simulink model "simulink_model"  (R2019b)
settings: Solver=ode15s  StartTime=0.0  StopTime=sim_time  FixedStep=1e-5
values from neighbouring files (symbols this model uses):
  A_t = 2000*eye(n)    [config_2R.m]    (also in config_3R.m)
  B2 = -Jinv    [computegains.m]
  B_t = eye(n)    [computegains.m]
  J = diag(rg.^2 .* Im_zz)    [model_2R.m]    (also in model_3R.m)
  Jinv = inv(J)    [computegains.m]
  K = diag(k_el)    [model_2R.m]    (also in model_3R.m)
  K1_t = lyap(A_t,Q_t)    [config_2R.m]    (also in config_3R.m)
  K2_t = 2000*eye(n)    [config_2R.m]    (also in config_3R.m)
  K_ctr = K_ctr*T_ctr    [computegains.m]
  K_ctr2 = -place(At,Bt,pls_ctr2)    [computegains.m]
  Ka_t = -10000*eye(n)    [config_2R.m]    (also in config_3R.m)
  n = 3    [simulation.m]
  x0 = [-pi/2 0   , 0 0 , -pi/2 0 , 0 0]    [config_2R.m]    (also in config_3R.m = [0 pi/2 0 , 0 0 0 , 0 pi/2 0 , 0 0 0])
  x0_hat = [x0(1) x0(2) , 0 0   , 0 0  ,   0 0]    [config_2R.m]    (also in config_3R.m = [x0(1) x0(2) x0(3) , 0 0 0 , 0 0 0 , 0 0 0])
undefined symbols (not defined in the file or in its folder): F_fun, Q1_fun, Q2_fun, Q_fun
settings Model: Creator=pietro  LastModifiedBy=pietro
settings SolverCC: MaxConsecutiveMinStep=10

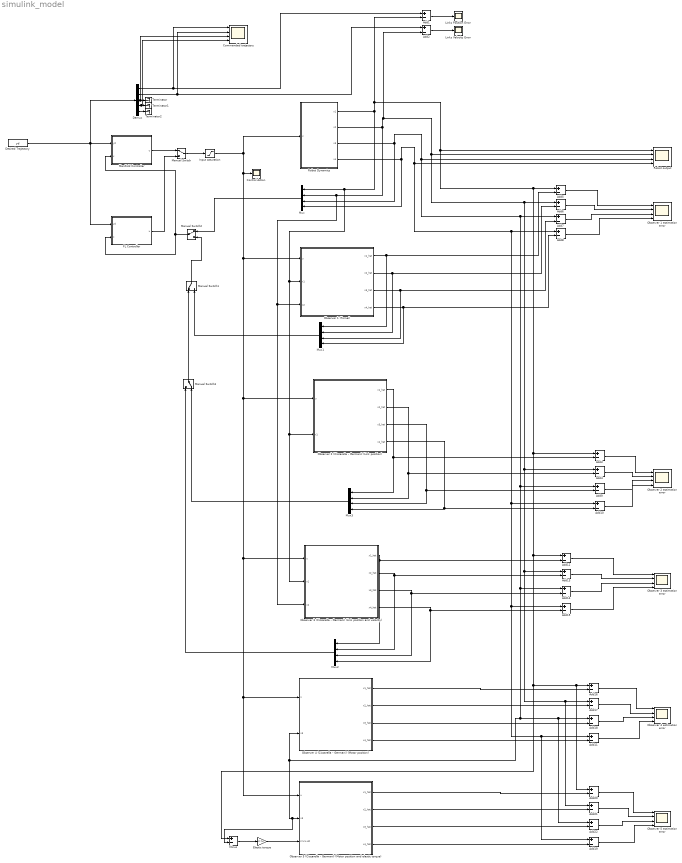
== system simulink_model ==
  Add{1..22} (22 alike) : Sum  Inputs=+-
  Commanded trajectory : Scope  NumInputPorts=4
  Control Action : Scope
  Demux : Demux  Outputs=[n;n;n;n;n]
  Desired Trajectory : FromWorkspace  VariableName=yd  SampleTime=0
  Elastic torque : Gain  Gain=K  Multiplication=Matrix(K*u) (u vector)
  FL Controller : Subsystem
  Input saturation : Saturate  UpperLimit=200  LowerLimit=-200
  Links Position Error : Scope
  Links Velocity Error : Scope
  Manifold Controller : Subsystem
  Manual Switch : ManualSwitch
  Manual Switch1 : ManualSwitch
  Manual Switch2 : ManualSwitch
  Manual Switch3 : ManualSwitch  CurrentSetting=0
  Minus : Sum  Inputs=+-
  Mux{,1..3} (4 alike) : Mux
  Observer 1 (Tomei) : Subsystem
  Observer 1 estimation error : Scope  NumInputPorts=4
  Observer 2 (Ciccarella - Germani) (Link position) : Subsystem
  Observer 2 estimation error : Scope  NumInputPorts=4
  Observer 3 (Ciccarella - Germani) (Link position and velocity) : Subsystem
  Observer 3 estimation error : Scope  NumInputPorts=4
  Observer 4 (Ciccarella - Germani) (Motor position) : Subsystem
  Observer 4 estimation error : Scope  NumInputPorts=4
  Observer 5 (Ciccarella - Germani) (Motor position and elastic torque) : Subsystem
  Observer 5 estimation error : Scope  NumInputPorts=4
  Robot Dynamics : Subsystem
  Robot output : Scope  NumInputPorts=4
  Terminator : Terminator
  Terminator1 : Terminator
  Terminator2 : Terminator
  wires:
  Desired Trajectory/1 -> FL Controller/1(yd), Demux/1, Manifold Controller/1(yd)
  Add5/1 -> Observer 1 estimation error/1
  Add6/1 -> Observer 1 estimation error/2
  Add7/1 -> Observer 1 estimation error/3
  Add8/1 -> Observer 1 estimation error/4
  Observer 1 (Tomei)/2(x2_hat) -> Mux1/2, Add6/2
  Observer 1 (Tomei)/3(x3_hat) -> Mux1/3, Add7/2
  Observer 1 (Tomei)/1(x1_hat) -> Mux1/1, Add5/2
  Observer 3 (Ciccarella - Germani) (Link position and velocity)/3(x3_hat) -> Mux2/3, Add14/2
  Observer 3 (Ciccarella - Germani) (Link position and velocity)/4(x4_hat) -> Mux2/4, Add15/2
  Add13/1 -> Observer 3 estimation error/2
  Add12/1 -> Observer 3 estimation error/1
  Add15/1 -> Observer 3 estimation error/4
  Add14/1 -> Observer 3 estimation error/3
  FL Controller/1(u) -> Manual Switch/2
  Manifold Controller/1(u) -> Manual Switch/1
  Manual Switch/1 -> Input saturation/1
  Mux/1 -> Manual Switch2/1
  Add1/1 -> Links Position Error/1
  Add2/1 -> Links Velocity Error/1
  Demux/1 -> Commanded trajectory/1, Add1/1
  Demux/2 -> Commanded trajectory/2, Add2/1
  Input saturation/1 -> Observer 5 (Ciccarella - Germani) (Motor position and elastic torque)/1(u), Observer 4 (Ciccarella - Germani) (Motor position)/1(u), Observer 3 (Ciccarella - Germani) (Link position and velocity)/1(u), Observer 2 (Ciccarella - Germani) (Link position)/1(u), Observer 1 (Tomei)/1(u), Control Action/1, Robot Dynamics/1(u)
  Demux/3 -> Commanded trajectory/3, Terminator/1
  Demux/4 -> Commanded trajectory/4, Terminator1/1
  Demux/5 -> Terminator2/1
  Observer 3 (Ciccarella - Germani) (Link position and velocity)/1(x1_hat) -> Mux2/1, Add12/2
  Observer 3 (Ciccarella - Germani) (Link position and velocity)/2(x2_hat) -> Mux2/2, Add13/2
  Observer 1 (Tomei)/4(x4_hat) -> Mux1/4, Add8/2
  Mux1/1 -> Manual Switch1/2
  Manual Switch1/1 -> Manual Switch2/2
  Manual Switch2/1 -> Manifold Controller/2(x), FL Controller/2(x)
  Manual Switch3/1 -> Manual Switch1/1
  Mux2/1 -> Manual Switch3/1
  Add10/1 -> Observer 2 estimation error/4
  Observer 2 (Ciccarella - Germani) (Link position)/1(x1_hat) -> Mux3/1, Add3/2
  Add9/1 -> Observer 2 estimation error/3
  Observer 2 (Ciccarella - Germani) (Link position)/2(x2_hat) -> Mux3/2, Add4/2
  Add4/1 -> Observer 2 estimation error/2
  Observer 2 (Ciccarella - Germani) (Link position)/4(x4_hat) -> Mux3/4, Add10/2
  Observer 2 (Ciccarella - Germani) (Link position)/3(x3_hat) -> Mux3/3, Add9/2
  Add3/1 -> Observer 2 estimation error/1
  Mux3/1 -> Manual Switch3/2
  Observer 4 (Ciccarella - Germani) (Motor position)/2(x2_hat) -> Add17/2
  Add16/1 -> Observer 4 estimation error/1
  Observer 4 (Ciccarella - Germani) (Motor position)/3(x3_hat) -> Add18/2
  Observer 4 (Ciccarella - Germani) (Motor position)/4(x4_hat) -> Add11/2
  Add18/1 -> Observer 4 estimation error/3
  Add11/1 -> Observer 4 estimation error/4
  Add17/1 -> Observer 4 estimation error/2
  Observer 4 (Ciccarella - Germani) (Motor position)/1(x1_hat) -> Add16/2
  Add22/1 -> Observer 5 estimation error/3
  Add21/1 -> Observer 5 estimation error/2
  Add20/1 -> Observer 5 estimation error/1
  Add19/1 -> Observer 5 estimation error/4
  Observer 5 (Ciccarella - Germani) (Motor position and elastic torque)/1(x1_hat) -> Add20/2
  Observer 5 (Ciccarella - Germani) (Motor position and elastic torque)/2(x2_hat) -> Add21/2
  Observer 5 (Ciccarella - Germani) (Motor position and elastic torque)/3(x3_hat) -> Add22/2
  Observer 5 (Ciccarella - Germani) (Motor position and elastic torque)/4(x4_hat) -> Add19/2
  Elastic torque/1 -> Observer 5 (Ciccarella - Germani) (Motor position and elastic torque)/3(K(x1-x3))
  Minus/1 -> Elastic torque/1
  Robot Dynamics/2(x2) -> Add2/2, Add4/1, Add21/1, Add17/1, Add13/1, Add6/1, Robot output/2, Observer 3 (Ciccarella - Germani) (Link position and velocity)/3(x2), Observer 1 (Tomei)/3(x2), Mux/2
  Robot Dynamics/1(x1) -> Add1/2, Add3/1, Minus/1, Add20/1, Add16/1, Add12/1, Add5/1, Robot output/1, Observer 2 (Ciccarella - Germani) (Link position)/2(x1), Observer 3 (Ciccarella - Germani) (Link position and velocity)/2(x1), Observer 1 (Tomei)/2(x1), Mux/1
  Robot Dynamics/3(x3) -> Add9/1, Minus/2, Observer 5 (Ciccarella - Germani) (Motor position and elastic torque)/2(x3), Observer 4 (Ciccarella - Germani) (Motor position)/2(x3), Add22/1, Add18/1, Add14/1, Add7/1, Robot output/3, Mux/3
  Robot Dynamics/4(x4) -> Add19/1, Add11/1, Add15/1, Add10/1, Add8/1, Robot output/4, Mux/4

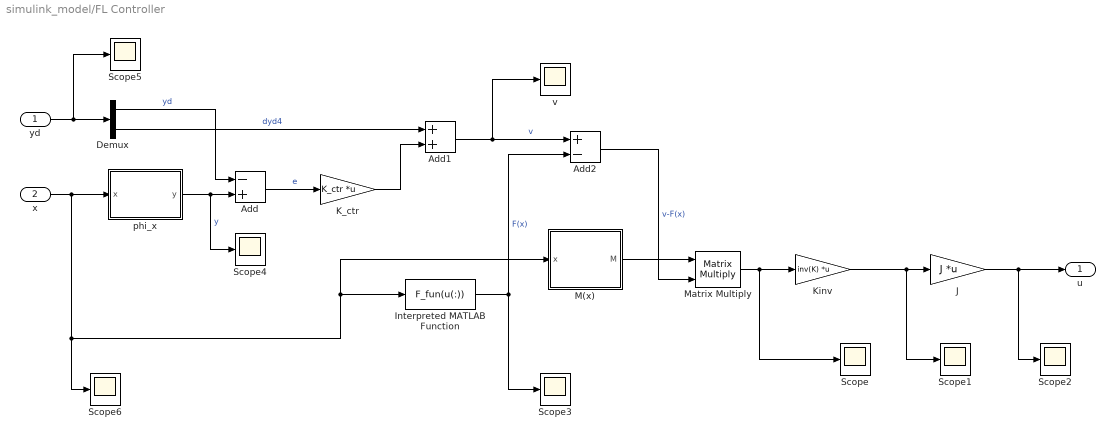
== system simulink_model/FL Controller ==
  yd : Inport
  x : Inport  Port=2
  Add : Sum  Inputs=-+
  Add1 : Sum
  Add2 : Sum  Inputs=+-
  Demux : Demux  Outputs=[4*n; n]
  Interpreted MATLAB Function : MATLABFcn  MATLABFcn=F_fun(u(:))  Output1D=off
  J : Gain  Gain=J  Multiplication=Matrix(K*u) (u vector)
  K_ctr : Gain  Gain=K_ctr  Multiplication=Matrix(K*u) (u vector)
  Kinv : Gain  Gain=inv(K)  Multiplication=Matrix(K*u) (u vector)
  M(x) : MATLAB Function  TreatAsAtomicUnit=on
  Matrix Multiply : Product  Inputs=**  Multiplication=Matrix(*)
  Scope{,1..6} (7 alike) : Scope
  phi_x : MATLAB Function  TreatAsAtomicUnit=on
  v : Scope
  u : Outport
  wires:
  x/1 -> Scope6/1, Interpreted MATLAB Function/1, M(x)/1(x), phi_x/1(x)
  phi_x/1(y) -> Scope4/1, Add/2  "y"
  yd/1 -> Scope5/1, Demux/1
  Add/1 -> K_ctr/1  "e"
  Demux/1 -> Add/1  "yd"
  Interpreted MATLAB Function/1 -> Add2/2, Scope3/1  "F(x)"
  J/1 -> Scope2/1, u/1
  Demux/2 -> Add1/1  "dyd4"
  Kinv/1 -> Scope1/1, J/1
  K_ctr/1 -> Add1/2
  Add1/1 -> v/1, Add2/1  "v"
  Matrix Multiply/1 -> Scope/1, Kinv/1
  Add2/1 -> Matrix Multiply/2  "v-F(x)"
  M(x)/1(M) -> Matrix Multiply/1

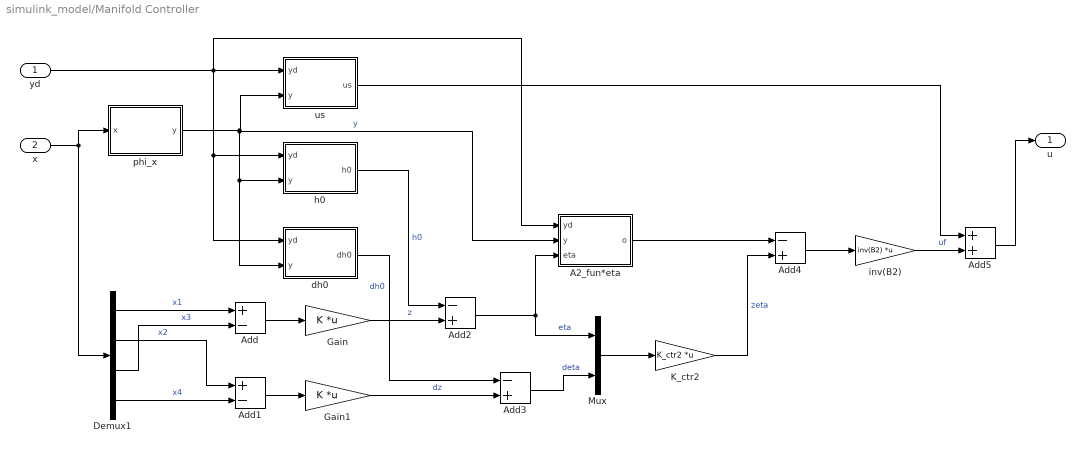
== system simulink_model/Manifold Controller ==
  yd : Inport
  x : Inport  Port=2
  A2_fun*eta : MATLAB Function  TreatAsAtomicUnit=on
  Add : Sum  Inputs=+-
  Add1 : Sum  Inputs=+-
  Add2 : Sum  Inputs=-+
  Add3 : Sum  Inputs=-+
  Add4 : Sum  Inputs=-+
  Add5 : Sum
  Demux1 : Demux  Outputs=[n;n;n;n]
  Gain : Gain  Gain=K  Multiplication=Matrix(K*u) (u vector)
  Gain1 : Gain  Gain=K  Multiplication=Matrix(K*u) (u vector)
  K_ctr2 : Gain  Gain=K_ctr2  Multiplication=Matrix(K*u) (u vector)
  Mux : Mux  Inputs=[n;n]
  dh0 : MATLAB Function  TreatAsAtomicUnit=on
  h0 : MATLAB Function  TreatAsAtomicUnit=on
  inv(B2) : Gain  Gain=inv(B2)  Multiplication=Matrix(K*u) (u vector)
  phi_x : MATLAB Function  TreatAsAtomicUnit=on
  us : MATLAB Function  TreatAsAtomicUnit=on
  u : Outport
  wires:
  x/1 -> Demux1/1, phi_x/1(x)
  yd/1 -> A2_fun*eta/1(yd), dh0/1(yd), h0/1(yd), us/1(yd)
  Add5/1 -> u/1
  Demux1/1 -> Add/1  "x1"
  Demux1/3 -> Add/2  "x3"
  Add/1 -> Gain/1
  Add1/1 -> Gain1/1
  Demux1/2 -> Add1/1  "x2"
  Demux1/4 -> Add1/2  "x4"
  phi_x/1(y) -> A2_fun*eta/2(y), dh0/2(y), h0/2(y), us/2(y)  "y"
  Gain/1 -> Add2/2  "z"
  h0/1(h0) -> Add2/1  "h0"
  Gain1/1 -> Add3/2  "dz"
  dh0/1(dh0) -> Add3/1  "dh0"
  Add2/1 -> A2_fun*eta/3(eta), Mux/1  "eta"
  Add3/1 -> Mux/2  "deta"
  Mux/1 -> K_ctr2/1
  K_ctr2/1 -> Add4/2  "zeta"
  A2_fun*eta/1(o) -> Add4/1
  Add4/1 -> inv(B2)/1
  inv(B2)/1 -> Add5/2  "uf"
  us/1(us) -> Add5/1

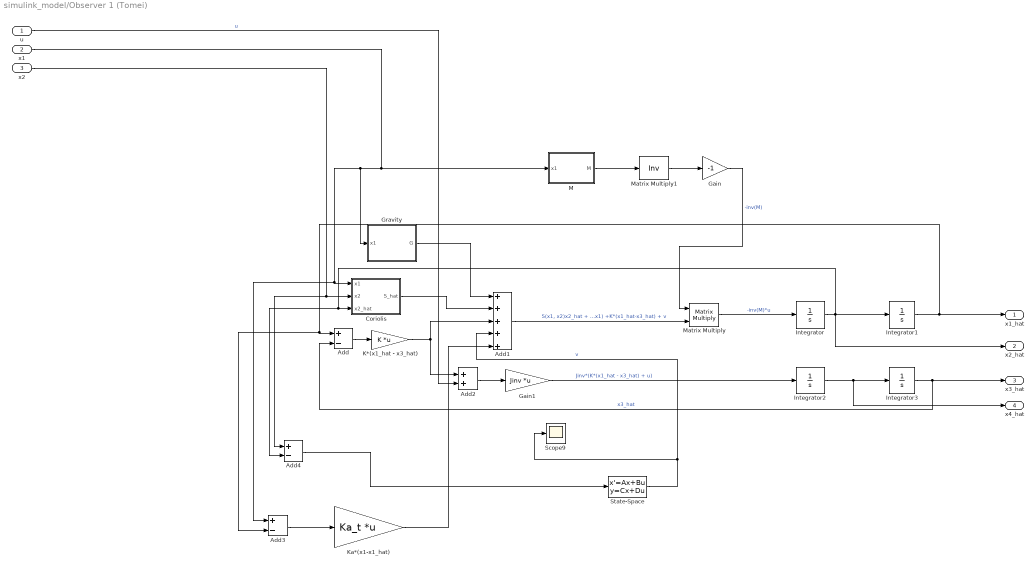
== system simulink_model/Observer 1 (Tomei) ==
  u : Inport
  x1 : Inport  Port=2
  x2 : Inport  Port=3
  Add : Sum  Inputs=+-
  Add1 : Sum  Inputs=+++++
  Add2 : Sum
  Add3 : Sum  Inputs=+-
  Add4 : Sum  Inputs=+-
  Coriolis : MATLAB Function  TreatAsAtomicUnit=on
  Gain : Gain  Gain=-1
  Gain1 : Gain  Gain=Jinv  Multiplication=Matrix(K*u) (u vector)
  Gravity : MATLAB Function  TreatAsAtomicUnit=on
  Integrator : Integrator  InitialCondition=x0_hat(n+1:2*n)
  Integrator1 : Integrator  InitialCondition=x0_hat(1:n)
  Integrator2 : Integrator  InitialCondition=x0_hat(3*n + 1:4*n)
  Integrator3 : Integrator  InitialCondition=x0_hat(2*n+1:3*n)
  K*(x1_hat - x3_hat) : Gain  Gain=K  Multiplication=Matrix(K*u) (u vector)
  Ka*(x1-x1_hat) : Gain  Gain=Ka_t  Multiplication=Matrix(K*u) (u vector)
  M : MATLAB Function  TreatAsAtomicUnit=on
  Matrix Multiply : Product  Multiplication=Matrix(*)
  Matrix Multiply1 : Product  Inputs=/  Multiplication=Matrix(*)
  Scope9 : Scope
  State-Space : StateSpace  A=-A_t  B=B_t  C=-K1_t  D=-K2_t  InitialCondition=0
  x1_hat : Outport
  x2_hat : Outport  Port=2
  x3_hat : Outport  Port=3
  x4_hat : Outport  Port=4
  wires:
  Add3/1 -> Ka*(x1-x1_hat)/1
  Add/1 -> K*(x1_hat - x3_hat)/1
  Add2/1 -> Gain1/1
  Integrator1/1 -> x1_hat/1, Add3/2, Add/1
  Add4/1 -> State-Space/1
  Integrator3/1 -> Add/2, x3_hat/1  "x3_hat"
  Ka*(x1-x1_hat)/1 -> Add1/5
  Gravity/1(G) -> Add1/1
  x1/1 -> M/1(x1), Gravity/1(x1), Add3/1, Coriolis/1(x1)
  x2/1 -> Add4/1, Coriolis/2(x2)
  State-Space/1 -> Add1/4, Scope9/1  "v"
  Add1/1 -> Matrix Multiply/2  "S(x1, x2)x2_hat + g(x1) +K*(x1_hat-x3_hat) + v"
  K*(x1_hat - x3_hat)/1 -> Add2/1, Add1/3
  Coriolis/1(S_hat) -> Add1/2
  u/1 -> Add2/2  "u"
  Gain1/1 -> Integrator2/1  "Jinv*(K*(x1_hat - x3_hat) + u)"
  Integrator/1 -> x2_hat/1, Add4/2, Coriolis/3(x2_hat), Integrator1/1
  Integrator2/1 -> x4_hat/1, Integrator3/1
  Matrix Multiply/1 -> Integrator/1  "-inv(M)*u"
  Gain/1 -> Matrix Multiply/1  "-inv(M)"
  M/1(M) -> Matrix Multiply1/1
  Matrix Multiply1/1 -> Gain/1

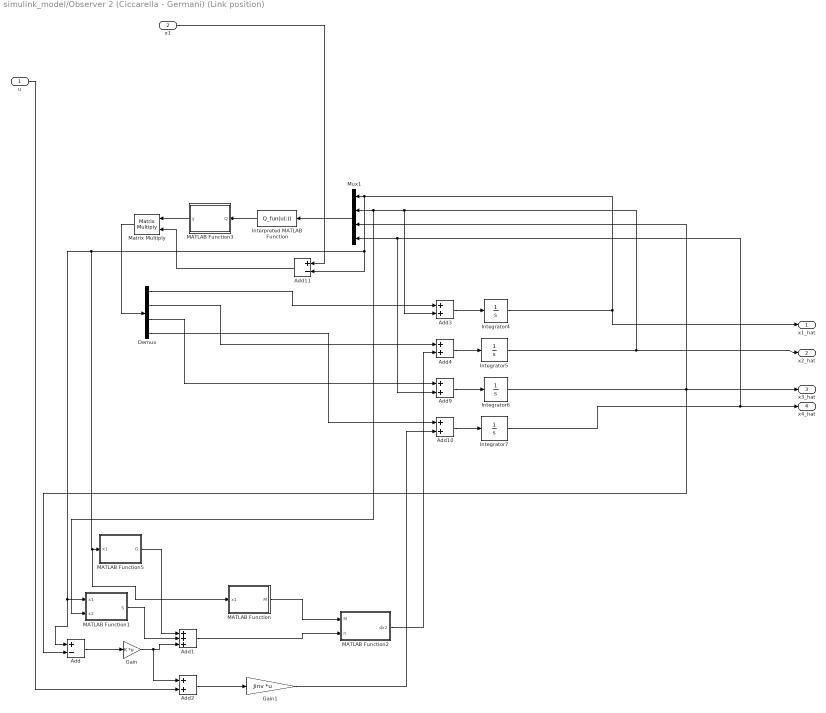
== system simulink_model/Observer 2 (Ciccarella - Germani) (Link position) ==
  u : Inport
  x1 : Inport  Port=2
  Add : Sum  Inputs=+-
  Add1 : Sum  Inputs=+++
  Add{2..4,9..10} (5 alike) : Sum
  Add11 : Sum  Inputs=+-
  Demux : Demux
  Gain : Gain  Gain=K  Multiplication=Matrix(K*u) (u vector)
  Gain1 : Gain  Gain=Jinv  Multiplication=Matrix(K*u) (u vector)
  Integrator4 : Integrator  InitialCondition=x0_hat(1:n)
  Integrator5 : Integrator  InitialCondition=x0_hat(n+1:2*n)  UpperSaturationLimit=5  LowerSaturationLimit=-5
  Integrator6 : Integrator  InitialCondition=x0_hat(2*n+1:3*n)
  Integrator7 : Integrator  InitialCondition=x0_hat(3*n + 1:4*n)  UpperSaturationLimit=5  LowerSaturationLimit=-5
  Interpreted MATLAB Function : MATLABFcn  MATLABFcn=Q_fun(u(:))  OutputDimensions=[4*n,4*n]  Output1D=off
  MATLAB Function : MATLAB Function  TreatAsAtomicUnit=on
  MATLAB Function1 : MATLAB Function  TreatAsAtomicUnit=on
  MATLAB Function2 : MATLAB Function  TreatAsAtomicUnit=on
  MATLAB Function3 : MATLAB Function  TreatAsAtomicUnit=on
  MATLAB Function5 : MATLAB Function  TreatAsAtomicUnit=on
  Matrix Multiply : Product  Multiplication=Matrix(*)
  Mux1 : Mux
  x1_hat : Outport
  x2_hat : Outport  Port=2
  x3_hat : Outport  Port=3
  x4_hat : Outport  Port=4
  wires:
  Integrator4/1 -> Mux1/1, Add11/2, MATLAB Function/1(x1), MATLAB Function5/1(x1), MATLAB Function1/1(x1), Add/1, x1_hat/1
  Integrator5/1 -> Mux1/2, MATLAB Function1/2(x2), Add3/2, x2_hat/1
  Integrator6/1 -> x3_hat/1, Mux1/3, Add/2
  Integrator7/1 -> x4_hat/1, Mux1/4, Add9/2
  Interpreted MATLAB Function/1 -> MATLAB Function3/1(Q)
  Demux/4 -> Add10/1
  Add/1 -> Gain/1
  Demux/3 -> Add9/1
  Mux1/1 -> Interpreted MATLAB Function/1
  Demux/1 -> Add3/1
  Add2/1 -> Gain1/1
  Add9/1 -> Integrator6/1
  Add11/1 -> Matrix Multiply/2
  MATLAB Function/1(M) -> MATLAB Function2/1(M)
  MATLAB Function2/1(dx2) -> Add4/2
  Demux/2 -> Add4/1
  MATLAB Function1/1(S) -> Add1/2
  MATLAB Function5/1(G) -> Add1/1
  Gain/1 -> Add1/3, Add2/1
  Add1/1 -> MATLAB Function2/2(n)
  x1/1 -> Add11/1
  Add10/1 -> Integrator7/1
  u/1 -> Add2/2
  MATLAB Function3/1(y) -> Matrix Multiply/1
  Matrix Multiply/1 -> Demux/1
  Gain1/1 -> Add10/2
  Add4/1 -> Integrator5/1
  Add3/1 -> Integrator4/1

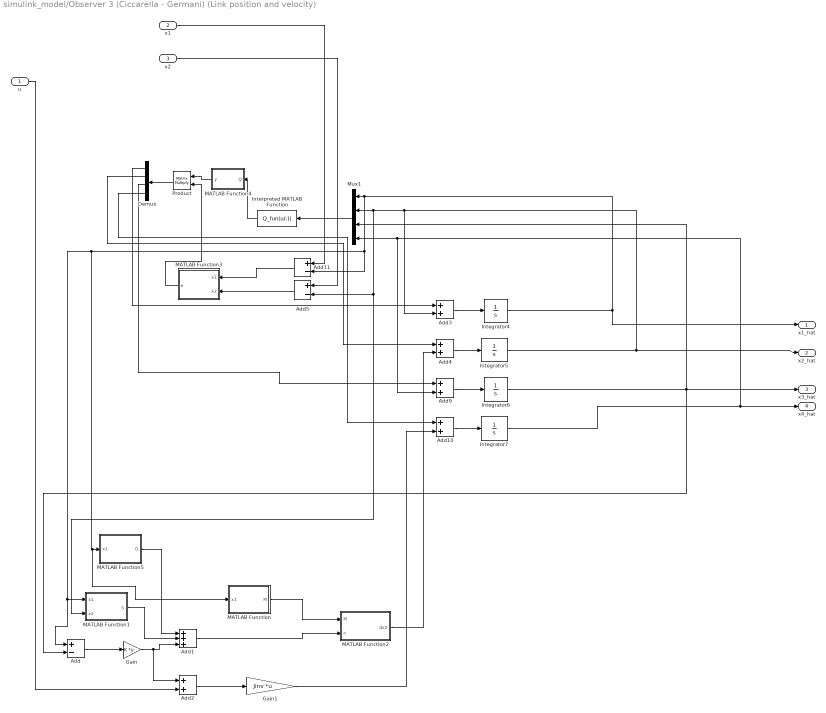
== system simulink_model/Observer 3 (Ciccarella - Germani) (Link position and velocity) ==
  u : Inport
  x1 : Inport  Port=2
  x2 : Inport  Port=3
  Add : Sum  Inputs=+-
  Add1 : Sum  Inputs=+++
  Add{2..4,9..10} (5 alike) : Sum
  Add11 : Sum  Inputs=+-
  Add5 : Sum  Inputs=+-
  Demux : Demux
  Gain : Gain  Gain=K  Multiplication=Matrix(K*u) (u vector)
  Gain1 : Gain  Gain=Jinv  Multiplication=Matrix(K*u) (u vector)
  Integrator4 : Integrator  InitialCondition=x0_hat(1:n)
  Integrator5 : Integrator  InitialCondition=x0_hat(n+1:2*n)  UpperSaturationLimit=5  LowerSaturationLimit=-5
  Integrator6 : Integrator  InitialCondition=x0_hat(2*n+1:3*n)
  Integrator7 : Integrator  InitialCondition=x0_hat(3*n + 1:4*n)  UpperSaturationLimit=5  LowerSaturationLimit=-5
  Interpreted MATLAB Function : MATLABFcn  MATLABFcn=Q_fun(u(:))  OutputDimensions=[4*n,4*n]  Output1D=off
  MATLAB Function : MATLAB Function  TreatAsAtomicUnit=on
  MATLAB Function1 : MATLAB Function  TreatAsAtomicUnit=on
  MATLAB Function2 : MATLAB Function  TreatAsAtomicUnit=on
  MATLAB Function3 : MATLAB Function  TreatAsAtomicUnit=on
  MATLAB Function4 : MATLAB Function  TreatAsAtomicUnit=on
  MATLAB Function5 : MATLAB Function  TreatAsAtomicUnit=on
  Mux1 : Mux
  Product : Product  Multiplication=Matrix(*)
  x1_hat : Outport
  x2_hat : Outport  Port=2
  x3_hat : Outport  Port=3
  x4_hat : Outport  Port=4
  wires:
  Add3/1 -> Integrator4/1
  Add4/1 -> Integrator5/1
  Gain1/1 -> Add10/2
  u/1 -> Add2/2
  Add10/1 -> Integrator7/1
  x1/1 -> Add11/1
  Add1/1 -> MATLAB Function2/2(n)
  Gain/1 -> Add2/1, Add1/3
  MATLAB Function5/1(G) -> Add1/1
  MATLAB Function1/1(S) -> Add1/2
  Demux/2 -> Add4/1
  MATLAB Function2/1(dx2) -> Add4/2
  MATLAB Function/1(M) -> MATLAB Function2/1(M)
  Add9/1 -> Integrator6/1
  Add2/1 -> Gain1/1
  Demux/1 -> Add3/1
  Mux1/1 -> Interpreted MATLAB Function/1
  Demux/3 -> Add9/1
  Add/1 -> Gain/1
  Demux/4 -> Add10/1
  Integrator7/1 -> Add9/2, Mux1/4, x4_hat/1
  Integrator6/1 -> Add/2, Mux1/3, x3_hat/1
  Integrator5/1 -> x2_hat/1, Add3/2, Add5/2, MATLAB Function1/2(x2), Mux1/2
  Integrator4/1 -> x1_hat/1, Add/1, MATLAB Function1/1(x1), MATLAB Function5/1(x1), MATLAB Function/1(x1), Add11/2, Mux1/1
  x2/1 -> Add5/1
  Add11/1 -> MATLAB Function3/1(x1)
  Add5/1 -> MATLAB Function3/2(x2)
  Product/1 -> Demux/1
  MATLAB Function3/1(e) -> Product/2
  MATLAB Function4/1(y) -> Product/1
  Interpreted MATLAB Function/1 -> MATLAB Function4/1(Q)

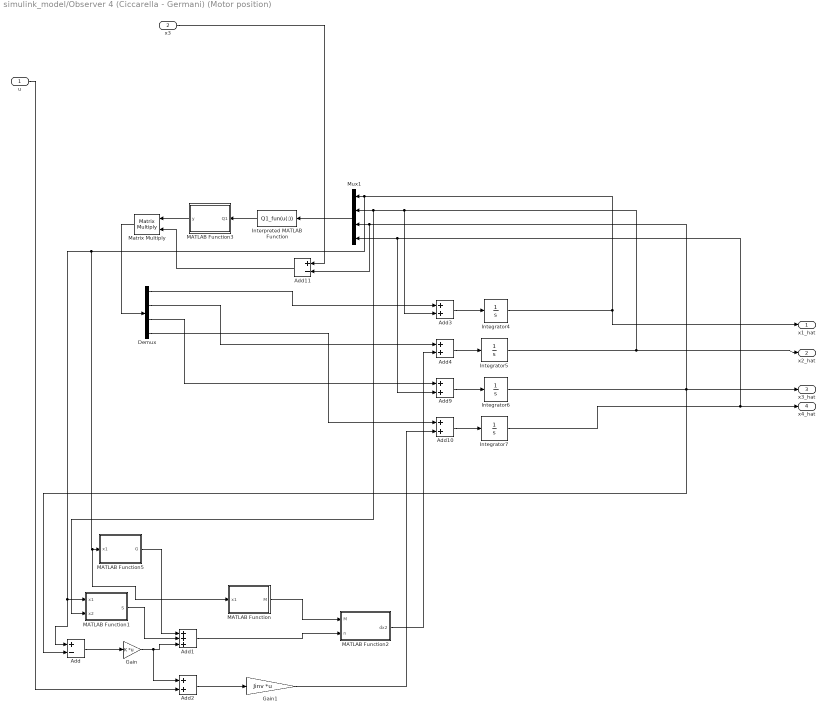
== system simulink_model/Observer 4 (Ciccarella - Germani) (Motor position) ==
  u : Inport
  x3 : Inport  Port=2
  Add : Sum  Inputs=+-
  Add1 : Sum  Inputs=+++
  Add{2..4,9..10} (5 alike) : Sum
  Add11 : Sum  Inputs=+-
  Demux : Demux
  Gain : Gain  Gain=K  Multiplication=Matrix(K*u) (u vector)
  Gain1 : Gain  Gain=Jinv  Multiplication=Matrix(K*u) (u vector)
  Integrator4 : Integrator  InitialCondition=x0_hat(1:n)
  Integrator5 : Integrator  InitialCondition=x0_hat(n+1:2*n)  UpperSaturationLimit=5  LowerSaturationLimit=-5
  Integrator6 : Integrator  InitialCondition=x0_hat(2*n+1:3*n)
  Integrator7 : Integrator  InitialCondition=x0_hat(3*n + 1:4*n)  UpperSaturationLimit=5  LowerSaturationLimit=-5
  Interpreted MATLAB Function : MATLABFcn  MATLABFcn=Q1_fun(u(:))  OutputDimensions=[4*n,4*n]  Output1D=off
  MATLAB Function : MATLAB Function  TreatAsAtomicUnit=on
  MATLAB Function1 : MATLAB Function  TreatAsAtomicUnit=on
  MATLAB Function2 : MATLAB Function  TreatAsAtomicUnit=on
  MATLAB Function3 : MATLAB Function  TreatAsAtomicUnit=on
  MATLAB Function5 : MATLAB Function  TreatAsAtomicUnit=on
  Matrix Multiply : Product  Multiplication=Matrix(*)
  Mux1 : Mux
  x1_hat : Outport
  x2_hat : Outport  Port=2
  x3_hat : Outport  Port=3
  x4_hat : Outport  Port=4
  wires:
  Integrator4/1 -> Mux1/1, MATLAB Function/1(x1), MATLAB Function5/1(x1), MATLAB Function1/1(x1), Add/1, x1_hat/1
  Integrator5/1 -> Mux1/2, MATLAB Function1/2(x2), Add3/2, x2_hat/1
  Integrator6/1 -> x3_hat/1, Add11/2, Mux1/3, Add/2
  Integrator7/1 -> x4_hat/1, Mux1/4, Add9/2
  Interpreted MATLAB Function/1 -> MATLAB Function3/1(Q1)
  Demux/4 -> Add10/1
  Add/1 -> Gain/1
  Demux/3 -> Add9/1
  Mux1/1 -> Interpreted MATLAB Function/1
  Demux/1 -> Add3/1
  Add2/1 -> Gain1/1
  Add9/1 -> Integrator6/1
  Add11/1 -> Matrix Multiply/2
  MATLAB Function/1(M) -> MATLAB Function2/1(M)
  MATLAB Function2/1(dx2) -> Add4/2
  Demux/2 -> Add4/1
  MATLAB Function1/1(S) -> Add1/2
  MATLAB Function5/1(G) -> Add1/1
  Gain/1 -> Add1/3, Add2/1
  Add1/1 -> MATLAB Function2/2(n)
  x3/1 -> Add11/1
  Add10/1 -> Integrator7/1
  u/1 -> Add2/2
  MATLAB Function3/1(y) -> Matrix Multiply/1
  Matrix Multiply/1 -> Demux/1
  Gain1/1 -> Add10/2
  Add4/1 -> Integrator5/1
  Add3/1 -> Integrator4/1

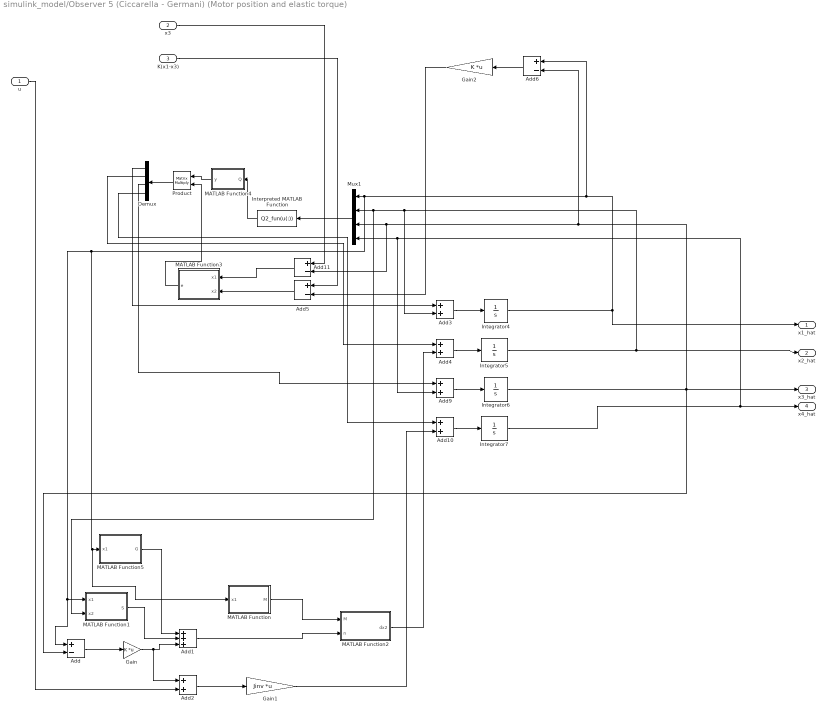
== system simulink_model/Observer 5 (Ciccarella - Germani) (Motor position and elastic torque) ==
  u : Inport
  x3 : Inport  Port=2
  K(x1-x3) : Inport  Port=3
  Add{,5..6,11} (4 alike) : Sum  Inputs=+-
  Add1 : Sum  Inputs=+++
  Add{2..4,9..10} (5 alike) : Sum
  Demux : Demux
  Gain : Gain  Gain=K  Multiplication=Matrix(K*u) (u vector)
  Gain1 : Gain  Gain=Jinv  Multiplication=Matrix(K*u) (u vector)
  Gain2 : Gain  Gain=K  Multiplication=Matrix(K*u) (u vector)
  Integrator4 : Integrator  InitialCondition=x0_hat(1:n)
  Integrator5 : Integrator  InitialCondition=x0_hat(n+1:2*n)  UpperSaturationLimit=5  LowerSaturationLimit=-5
  Integrator6 : Integrator  InitialCondition=x0_hat(2*n+1:3*n)
  Integrator7 : Integrator  InitialCondition=x0_hat(3*n + 1:4*n)  UpperSaturationLimit=5  LowerSaturationLimit=-5
  Interpreted MATLAB Function : MATLABFcn  MATLABFcn=Q2_fun(u(:))  OutputDimensions=[4*n,4*n]  Output1D=off
  MATLAB Function : MATLAB Function  TreatAsAtomicUnit=on
  MATLAB Function1 : MATLAB Function  TreatAsAtomicUnit=on
  MATLAB Function2 : MATLAB Function  TreatAsAtomicUnit=on
  MATLAB Function3 : MATLAB Function  TreatAsAtomicUnit=on
  MATLAB Function4 : MATLAB Function  TreatAsAtomicUnit=on
  MATLAB Function5 : MATLAB Function  TreatAsAtomicUnit=on
  Mux1 : Mux
  Product : Product  Multiplication=Matrix(*)
  x1_hat : Outport
  x2_hat : Outport  Port=2
  x3_hat : Outport  Port=3
  x4_hat : Outport  Port=4
  wires:
  Add3/1 -> Integrator4/1
  Add4/1 -> Integrator5/1
  Gain1/1 -> Add10/2
  u/1 -> Add2/2
  Add10/1 -> Integrator7/1
  x3/1 -> Add11/1
  Add1/1 -> MATLAB Function2/2(n)
  Gain/1 -> Add2/1, Add1/3
  MATLAB Function5/1(G) -> Add1/1
  MATLAB Function1/1(S) -> Add1/2
  Demux/2 -> Add4/1
  MATLAB Function2/1(dx2) -> Add4/2
  MATLAB Function/1(M) -> MATLAB Function2/1(M)
  Add9/1 -> Integrator6/1
  Add2/1 -> Gain1/1
  Demux/1 -> Add3/1
  Mux1/1 -> Interpreted MATLAB Function/1
  Demux/3 -> Add9/1
  Add/1 -> Gain/1
  Demux/4 -> Add10/1
  Integrator7/1 -> Add9/2, Mux1/4, x4_hat/1
  Integrator6/1 -> Add/2, Add6/2, Add11/2, Mux1/3, x3_hat/1
  Integrator5/1 -> x2_hat/1, Add3/2, MATLAB Function1/2(x2), Mux1/2
  Integrator4/1 -> x1_hat/1, Add6/1, Add/1, MATLAB Function1/1(x1), MATLAB Function5/1(x1), MATLAB Function/1(x1), Mux1/1
  K(x1-x3)/1 -> Add5/1
  Add11/1 -> MATLAB Function3/1(x1)
  Add5/1 -> MATLAB Function3/2(x2)
  Product/1 -> Demux/1
  MATLAB Function3/1(e) -> Product/2
  MATLAB Function4/1(y) -> Product/1
  Interpreted MATLAB Function/1 -> MATLAB Function4/1(Q)
  Add6/1 -> Gain2/1
  Gain2/1 -> Add5/2

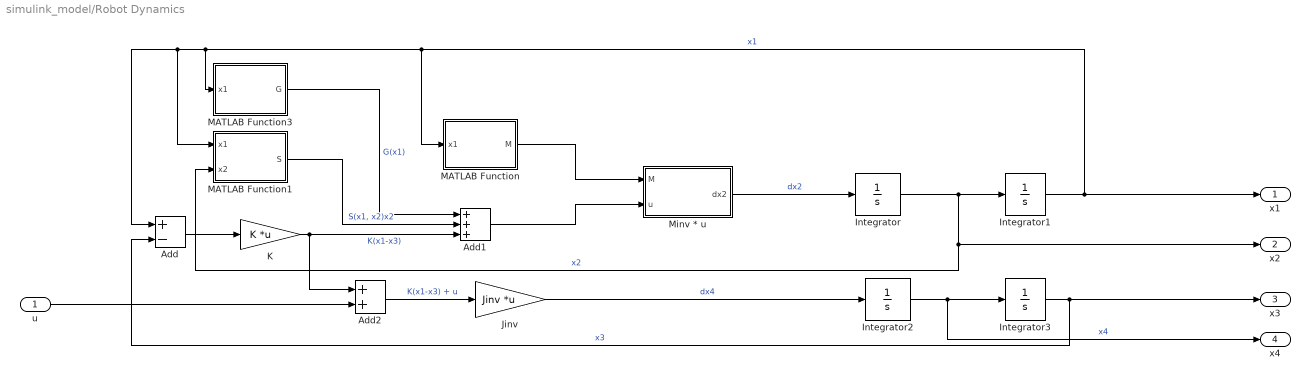
== system simulink_model/Robot Dynamics ==
  u : Inport
  Add : Sum  Inputs=+-
  Add1 : Sum  Inputs=+++
  Add2 : Sum
  Integrator : Integrator  InitialCondition=x0(n+1:2*n)
  Integrator1 : Integrator  InitialCondition=x0(1:n)
  Integrator2 : Integrator  InitialCondition=x0(3*n + 1:4*n)
  Integrator3 : Integrator  InitialCondition=x0(2*n+1:3*n)
  Jinv : Gain  Gain=Jinv  Multiplication=Matrix(K*u) (u vector)
  K : Gain  Gain=K  Multiplication=Matrix(K*u) (u vector)
  MATLAB Function : MATLAB Function  TreatAsAtomicUnit=on
  MATLAB Function1 : MATLAB Function  TreatAsAtomicUnit=on
  MATLAB Function3 : MATLAB Function  TreatAsAtomicUnit=on
  Minv * u : MATLAB Function  TreatAsAtomicUnit=on
  x1 : Outport
  x2 : Outport  Port=2
  x3 : Outport  Port=3
  x4 : Outport  Port=4
  wires:
  MATLAB Function1/1(S) -> Add1/2  "S(x1, x2)x2"
  Add1/1 -> Minv * u/2(u)
  MATLAB Function/1(M) -> Minv * u/1(M)
  u/1 -> Add2/2
  Integrator3/1 -> x3/1, Add/2  "x3"
  Integrator/1 -> x2/1, MATLAB Function1/2(x2), Integrator1/1  "x2"
  Add/1 -> K/1
  Add2/1 -> Jinv/1  "K(x1-x3) + u"
  Integrator2/1 -> x4/1, Integrator3/1  "x4"
  K/1 -> Add2/1, Add1/3  "K(x1-x3)"
  Integrator1/1 -> x1/1, MATLAB Function/1(x1), MATLAB Function3/1(x1), MATLAB Function1/1(x1), Add/1  "x1"
  Jinv/1 -> Integrator2/1  "dx4"
  MATLAB Function3/1(G) -> Add1/1  "G(x1)"
  Minv * u/1(dx2) -> Integrator/1  "dx2"

== matlab function simulink_model/Robot Dynamics/MATLAB Function1 ==
  data: x1 input; S output size=n; x2 input
function S = fcn(x1,x2)
S = S_fun(x1,x2)*x2;

== matlab function simulink_model/Robot Dynamics/MATLAB Function ==
  data: x1 input; M output size=[n,n]
function M = fcn(x1)
M = M_fun(x1);

== matlab function simulink_model/Observer 1 (Tomei)/M ==
  data: x1 input; M output size=[n,n]
function M = Minv(x1)
M = M_fun(x1);

== matlab function simulink_model/Observer 1 (Tomei)/Coriolis ==
  data: x1 input; x2 input; S_hat output size=n; x2_hat input
function S_hat = S(x1,x2,x2_hat)
S_hat = S_fun(x1,x2)*x2_hat;

== matlab function simulink_model/Robot Dynamics/Minv * u ==
  data: M input; dx2 output size=n; u input
function dx2 = fcn(M, u)
dx2 = -M\u;

== matlab function simulink_model/Observer 3 (Ciccarella - Germani) (Link position and velocity)/MATLAB Function ==
  data: x1 input; M output size=[n,n]
function M = fcn(x1)
M = M_fun(x1);

== matlab function simulink_model/Observer 3 (Ciccarella - Germani) (Link position and velocity)/MATLAB Function5 ==
  data: x1 input; G output size=n
function G = fcn(x1)
G = G_fun(x1);

== matlab function simulink_model/Manifold Controller/us ==
  data: yd input; us output; y input
function us = fcn(yd, y)
us = us_fun(y, yd);

== matlab function simulink_model/Observer 3 (Ciccarella - Germani) (Link position and velocity)/MATLAB Function1 ==
  data: x1 input; S output size=n; x2 input
function S = S(x1,x2)
S = S_fun(x1,x2)*x2;

== matlab function simulink_model/Observer 3 (Ciccarella - Germani) (Link position and velocity)/MATLAB Function2 ==
  data: M input; dx2 output size=n; n input
function dx2 = fcn(M,n)
dx2 = -M\n;

== matlab function simulink_model/Observer 3 (Ciccarella - Germani) (Link position and velocity)/MATLAB Function3 ==
  data: e output; x1 input; x2 input
function e = fcn(x1, x2)
[n,~] = size(x2);
e = zeros(2*n,1);
for i = 1 : n
    idx = 2*i - 1;
    e(idx,1) = x1(i);
    e(idx+1,1) = x2(i);
end

== matlab function simulink_model/Observer 3 (Ciccarella - Germani) (Link position and velocity)/MATLAB Function4 ==
  data: y output; Q input; K_obs_2 parameter
function y = fcn(Q, K_obs_2)
y = pinv(Q)*K_obs_2;

== matlab function simulink_model/FL Controller/phi_x ==
  data: x input size=4*n; y output
function y = fcn(x)
y = phix_fun(x);

== matlab function simulink_model/FL Controller/M(x) ==
  data: x input size=4*n; M output size=[n n]; n parameter size=1; J parameter; K parameter
function M = fcn(x, n, J, K)
x1 = x(1:n);
M = M_fun(x1);

== matlab function simulink_model/Observer 2 (Ciccarella - Germani) (Link position)/MATLAB Function ==
  data: x1 input; M output size=[n,n]
function M = fcn(x1)
M = M_fun(x1);

== matlab function simulink_model/Observer 2 (Ciccarella - Germani) (Link position)/MATLAB Function1 ==
  data: x1 input; S output size=n; x2 input
function S = S(x1,x2)
S = S_fun(x1,x2)*x2;

== matlab function simulink_model/Manifold Controller/h0 ==
  data: yd input; h0 output; y input
function h0 = fcn(yd, y)
h0 = h0_fun(y, yd);

== matlab function simulink_model/Manifold Controller/phi_x ==
  data: x input size=4*n; y output
function y = fcn(x)
y = phix_fun(x);

== matlab function simulink_model/Manifold Controller/dh0 ==
  data: yd input; dh0 output; y input
function dh0 = fcn(yd, y)
dh0 = dh0_fun(y, yd);

== matlab function simulink_model/Manifold Controller/A2_fun*eta ==
  data: yd input; o output; y input; eta input
function o = fcn(yd, y, eta)
o = A2_fun(y,yd)*eta;

== matlab function simulink_model/Robot Dynamics/MATLAB Function3 ==
  data: x1 input; G output size=n
function G = fcn(x1)
G = G_fun(x1);

== matlab function simulink_model/Observer 1 (Tomei)/Gravity ==
  data: x1 input; G output size=n
function G = fcn(x1)
G = G_fun(x1);

== matlab function simulink_model/Observer 2 (Ciccarella - Germani) (Link position)/MATLAB Function2 ==
  data: M input; dx2 output size=n; n input
function dx2 = fcn(M,n)
dx2 = -M\n;

== matlab function simulink_model/Observer 2 (Ciccarella - Germani) (Link position)/MATLAB Function3 ==
  data: Q input; y output size=[4*n,n]; K_obs_1 parameter
function y = fcn(Q,K_obs_1)
y = pinv(Q)*K_obs_1;

== matlab function simulink_model/Observer 2 (Ciccarella - Germani) (Link position)/MATLAB Function5 ==
  data: x1 input; G output size=n
function G = fcn(x1)
G = G_fun(x1);

== matlab function simulink_model/Observer 4 (Ciccarella - Germani) (Motor position)/MATLAB Function ==
  data: x1 input; M output size=[n,n]
function M = fcn(x1)
M = M_fun(x1);

== matlab function simulink_model/Observer 4 (Ciccarella - Germani) (Motor position)/MATLAB Function1 ==
  data: x1 input; S output size=n; x2 input
function S = S(x1,x2)
S = S_fun(x1,x2)*x2;

== matlab function simulink_model/Observer 4 (Ciccarella - Germani) (Motor position)/MATLAB Function2 ==
  data: M input; dx2 output size=n; n input
function dx2 = fcn(M,n)
dx2 = -M\n;

== matlab function simulink_model/Observer 4 (Ciccarella - Germani) (Motor position)/MATLAB Function3 ==
  data: Q1 input; y output size=[4*n,n]; K_obs_1 parameter
function y = fcn(Q1,K_obs_1)
y = pinv(Q1)*K_obs_1;

== matlab function simulink_model/Observer 4 (Ciccarella - Germani) (Motor position)/MATLAB Function5 ==
  data: x1 input; G output size=n
function G = fcn(x1)
G = G_fun(x1);

== matlab function simulink_model/Observer 5 (Ciccarella - Germani) (Motor position and elastic torque)/MATLAB Function ==
  data: x1 input; M output size=[n,n]
function M = fcn(x1)
M = M_fun(x1);

== matlab function simulink_model/Observer 5 (Ciccarella - Germani) (Motor position and elastic torque)/MATLAB Function1 ==
  data: x1 input; S output size=n; x2 input
function S = S(x1,x2)
S = S_fun(x1,x2)*x2;

== matlab function simulink_model/Observer 5 (Ciccarella - Germani) (Motor position and elastic torque)/MATLAB Function2 ==
  data: M input; dx2 output size=n; n input
function dx2 = fcn(M,n)
dx2 = -M\n;

== matlab function simulink_model/Observer 5 (Ciccarella - Germani) (Motor position and elastic torque)/MATLAB Function3 ==
  data: e output; x1 input; x2 input
function e = fcn(x1, x2)
e = [x1;x2];

== matlab function simulink_model/Observer 5 (Ciccarella - Germani) (Motor position and elastic torque)/MATLAB Function4 ==
  data: y output; Q input; K_obs_3 parameter
function y = fcn(Q, K_obs_3)
y = pinv(Q)*K_obs_3;

== matlab function simulink_model/Observer 5 (Ciccarella - Germani) (Motor position and elastic torque)/MATLAB Function5 ==
  data: x1 input; G output size=n
function G = fcn(x1)
G = G_fun(x1);
